simulink model "global_noise"  (R2023a)
settings: Solver=VariableStepAuto  StartTime=0.0  StopTime=10  RelTol=1e-3
values from neighbouring files (symbols this model uses):
  Ad = [0 0 0 0 0 0 ... (first row only)    [Project_globale.m]    (also in Project_locale.m)
  Ai = A0    [Project_globale.m]    (also in Project_locale.m)
  Bi = [ 0 ; -9.9453]    [Project_globale.m]    (also in Project_locale.m)
  c = 10/2*min(real(lambda_g))    [Project_globale.m]    (also in Project_locale.m)
  Ci = [708.27 0]    [Project_globale.m]    (also in Project_locale.m)
  F = P*Ci'*R^-1    [Project_globale.m]
  G = diag([1 0 0 0 0 0])    [Project_globale.m]    (also in Project_locale.m)
  K = R^-1*Bi'*P    [Project_globale.m]    (also in Project_locale.m)
  L0 = place(Ai',Ci',[0 -3])'    [Project_globale.m]
  x0 = [3,1]    [Project_globale.m]    (also in Project_locale.m)
settings Model: Creator=Giulia  LastModifiedBy=Giulia

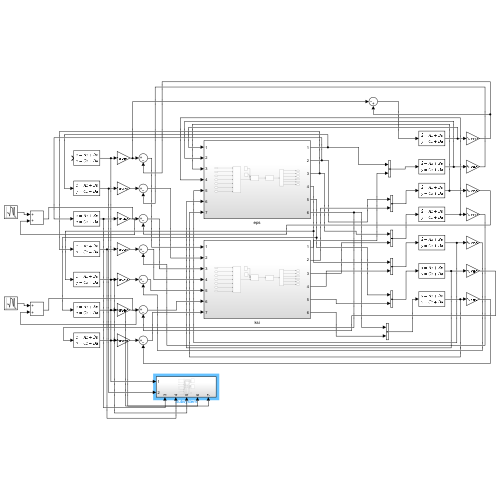
[thumbnail: Simulink's stored preview of the top-level diagram]
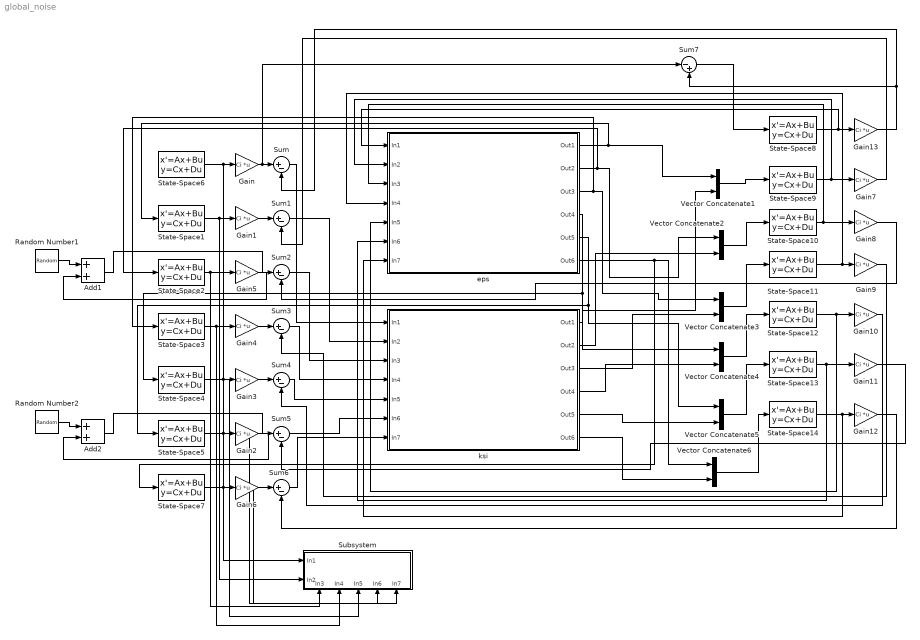
== system global_noise ==
  Add1 : Sum
  Add2 : Sum
  Gain{,1..13} (14 alike) : Gain  Gain=Ci  Multiplication=Matrix(K*u) (u vector)
  Random Number1 : RandomNumber  Variance=10000  SampleTime=0.1
  Random Number2 : RandomNumber  Variance=10000  SampleTime=0.1
  State-Space{1..5,7} (6 alike) : StateSpace  A=Ai  B=c*Bi*K  C=eye(2)  D=zeros(2,2)  InitialCondition=x0  ParameterTunability=Optimized
  State-Space{9..14} (6 alike) : StateSpace  A=Ai  B=[c*Bi*K,-c*F]  C=eye(2)  D=zeros(2,3)  InitialCondition=x0  ParameterTunability=Optimized
  State-Space6 : StateSpace  A=Ai  B=Bi  C=eye(2)  D=zeros(2,1)  InitialCondition=x0  ParameterTunability=Optimized
  State-Space8 : StateSpace  A=Ai  B=-L0  C=eye(2)  D=zeros(2,1)  InitialCondition=x0  ParameterTunability=Optimized
  Subsystem : Subsystem
      settings: PortSchema="{\"entries\":[{\"content\":{\"sides\":[{\"content\":{\"connectorIds\":[\"In1\",\"In2\"]},\"type\":\"ConnectorPlacement.EquallySpacedRectSide\",\"uuid\":\"e5690f60-dfa3-4d24-845c-eb19d446c7ee\"},{\"content\":{\"side\":\"RIGHT\"},\"type\":\"ConnectorPlacement.EquallySpacedRectSide\",\"uuid\":\"a41d9e4a-267d-44ba-a380-b8d8ea4e3cb9\"},{\"content\":{\"side\":\"TOP\"},\"type\":\"ConnectorPlacement.EquallySpacedRectSide\",\"uuid\":\"990e4c72-4654-4e9a-98e4-634db6676fa3\"},{\"content\":{\"connectorIds\":[\"In3\",\"In4\",\"In5\",\"In6\",\"In7\"],\"side\":\"BOTTOM\"},\"type\":\"ConnectorPlacement.EquallySpacedRectSide\",\"uuid\":\"e75a7693-b495-4998-ab10-28f33e3d4652\"}]},\"type\":\"ConnectorPlacement.EquallySpacedConnector\",\"uuid\":\"cc17a25f-dba8-4ee4-98f7-88763bf16359\"}],\"packageUris\":[\"http://schema.mathworks.com/mf0/Connector/R2020b\"],\"version\":\"1.0\"}"
  Sum{,1..6} (7 alike) : Sum  Inputs=|+-
  Sum7 : Sum  Inputs=|-+
  Vector Concatenate{1..6} (6 alike) : Concatenate
  eps : Subsystem
  ksi : Subsystem
  wires:
  ksi/1(Out1) -> Vector Concatenate1/2
  Sum6/1 -> ksi/7(In7)
  Gain/1 -> Sum7/1, Sum/1
  Sum3/1 -> ksi/4(In4)
  Sum2/1 -> ksi/3(In3)
  Sum5/1 -> ksi/6(In6)
  Gain7/1 -> Sum1/2
  Gain9/1 -> Sum3/2
  Sum4/1 -> ksi/5(In5)
  Gain8/1 -> Sum2/2
  Gain13/1 -> Sum7/2, Sum/2
  Gain10/1 -> Sum4/2
  Vector Concatenate6/1 -> State-Space14/1
  Vector Concatenate3/1 -> State-Space11/1
  ksi/2(Out2) -> Vector Concatenate2/2
  ksi/4(Out4) -> Vector Concatenate4/2
  Vector Concatenate2/1 -> State-Space10/1
  ksi/6(Out6) -> Vector Concatenate6/2
  eps/4(Out4) -> State-Space4/1, Vector Concatenate4/1
  eps/5(Out5) -> State-Space5/1, Vector Concatenate5/1
  Gain11/1 -> Sum5/2
  eps/6(Out6) -> State-Space7/1, Vector Concatenate6/1
  State-Space12/1 -> eps/5(In5), Gain10/1
  ksi/3(Out3) -> Vector Concatenate3/2
  eps/2(Out2) -> State-Space2/1, Vector Concatenate2/1
  State-Space8/1 -> eps/1(In1), Gain13/1
  eps/1(Out1) -> State-Space1/1, Vector Concatenate1/1
  State-Space11/1 -> eps/4(In4), Gain9/1
  State-Space13/1 -> eps/6(In6), Gain11/1
  State-Space4/1 -> Subsystem/5(In5), Gain3/1
  Vector Concatenate4/1 -> State-Space12/1
  Gain3/1 -> Sum4/1
  Sum/1 -> ksi/1(In1)
  Sum1/1 -> ksi/2(In2)
  ksi/5(Out5) -> Vector Concatenate5/2
  Vector Concatenate5/1 -> State-Space13/1
  State-Space3/1 -> Subsystem/4(In4), Gain4/1
  Gain1/1 -> Sum1/1
  eps/3(Out3) -> State-Space3/1, Vector Concatenate3/1
  Vector Concatenate1/1 -> State-Space9/1
  State-Space1/1 -> Subsystem/2(In2), Gain1/1
  State-Space6/1 -> Subsystem/1(In1), Gain/1
  State-Space9/1 -> eps/2(In2), Gain7/1
  Gain12/1 -> Sum6/2
  Sum7/1 -> State-Space8/1
  State-Space14/1 -> eps/7(In7), Gain12/1
  State-Space10/1 -> Gain8/1, eps/3(In3)
  State-Space2/1 -> Subsystem/3(In3), Gain5/1
  State-Space5/1 -> Subsystem/6(In6), Gain2/1
  Gain4/1 -> Sum3/1
  State-Space7/1 -> Subsystem/7(In7), Gain6/1
  Random Number1/1 -> Add1/1
  Add1/1 -> Sum2/1
  Gain5/1 -> Add1/2
  Random Number2/1 -> Add2/1
  Gain2/1 -> Add2/2
  Add2/1 -> Sum5/1
  Gain6/1 -> Sum6/1

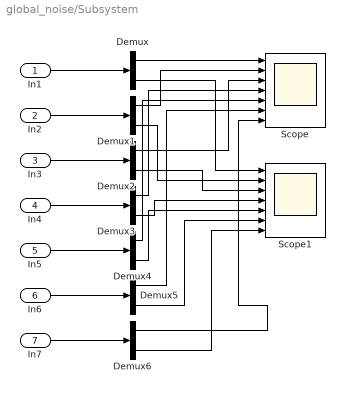
== system global_noise/Subsystem ==
  In1 : Inport
  In2 : Inport  Port=2
  In3 : Inport  Port=3
  In4 : Inport  Port=4
  In5 : Inport  Port=5
  In6 : Inport  Port=6
  In7 : Inport  Port=7
  Demux{,1..6} (7 alike) : Demux  Outputs=2
  Scope : Scope  NumInputPorts=7
  Scope1 : Scope  NumInputPorts=7
  wires:
  In1/1 -> Demux/1
  In2/1 -> Demux1/1
  In3/1 -> Demux2/1
  In4/1 -> Demux3/1
  In5/1 -> Demux4/1
  In6/1 -> Demux5/1
  In7/1 -> Demux6/1
  Demux/1 -> Scope/1
  Demux1/1 -> Scope/2
  Demux2/1 -> Scope/3
  Demux3/1 -> Scope/4
  Demux4/1 -> Scope/5
  Demux5/1 -> Scope/6
  Demux6/1 -> Scope/7
  Demux/2 -> Scope1/1
  Demux1/2 -> Scope1/2
  Demux2/2 -> Scope1/3
  Demux3/2 -> Scope1/4
  Demux4/2 -> Scope1/5
  Demux5/2 -> Scope1/6
  Demux6/2 -> Scope1/7

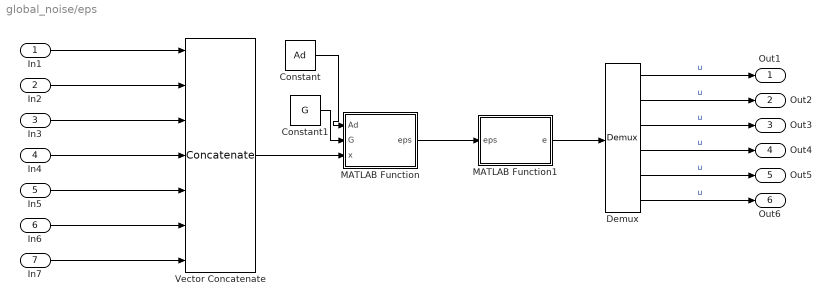
== system global_noise/eps ==
  In1 : Inport
  In2 : Inport  Port=2
  In3 : Inport  Port=3
  In4 : Inport  Port=4
  In5 : Inport  Port=5
  In6 : Inport  Port=6
  In7 : Inport  Port=7
  Constant : Constant  Value=Ad
  Constant1 : Constant  Value=G
  Demux : Demux  Outputs=size(Ad,1)
  MATLAB Function : MATLAB Function  TreatAsAtomicUnit=on
  MATLAB Function1 : MATLAB Function  TreatAsAtomicUnit=on
  Vector Concatenate : Concatenate  NumInputs=7  Mode=Multidimensional array  ConcatenateDimension=2
  Out1 : Outport
  Out2 : Outport  Port=2
  Out3 : Outport  Port=3
  Out4 : Outport  Port=4
  Out5 : Outport  Port=5
  Out6 : Outport  Port=6
  wires:
  MATLAB Function1/1(e) -> Demux/1
  Constant/1 -> MATLAB Function/1(Ad)
  MATLAB Function/1(eps) -> MATLAB Function1/1(eps)
  Constant1/1 -> MATLAB Function/2(G)
  Vector Concatenate/1 -> MATLAB Function/3(x)
  In1/1 -> Vector Concatenate/1
  In2/1 -> Vector Concatenate/2
  In3/1 -> Vector Concatenate/3
  In4/1 -> Vector Concatenate/4
  In5/1 -> Vector Concatenate/5
  In6/1 -> Vector Concatenate/6
  In7/1 -> Vector Concatenate/7
  Demux/1 -> Out1/1  "u"
  Demux/2 -> Out2/1  "u"
  Demux/3 -> Out3/1  "u"
  Demux/4 -> Out4/1  "u"
  Demux/5 -> Out5/1  "u"
  Demux/6 -> Out6/1  "u"

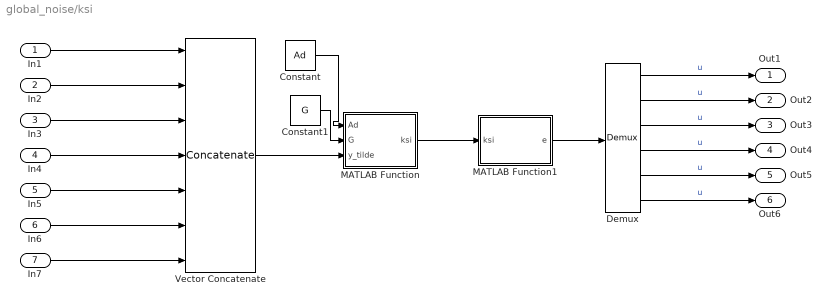
== system global_noise/ksi ==
  In1 : Inport
  In2 : Inport  Port=2
  In3 : Inport  Port=3
  In4 : Inport  Port=4
  In5 : Inport  Port=5
  In6 : Inport  Port=6
  In7 : Inport  Port=7
  Constant : Constant  Value=Ad
  Constant1 : Constant  Value=G
  Demux : Demux  Outputs=size(Ad,1)
  MATLAB Function : MATLAB Function  TreatAsAtomicUnit=on
  MATLAB Function1 : MATLAB Function  TreatAsAtomicUnit=on
  Vector Concatenate : Concatenate  NumInputs=7  Mode=Multidimensional array  ConcatenateDimension=2
  Out1 : Outport
  Out2 : Outport  Port=2
  Out3 : Outport  Port=3
  Out4 : Outport  Port=4
  Out5 : Outport  Port=5
  Out6 : Outport  Port=6
  wires:
  MATLAB Function1/1(e) -> Demux/1
  Constant/1 -> MATLAB Function/1(Ad)
  MATLAB Function/1(ksi) -> MATLAB Function1/1(ksi)
  Constant1/1 -> MATLAB Function/2(G)
  Vector Concatenate/1 -> MATLAB Function/3(y_tilde)
  In1/1 -> Vector Concatenate/1
  In2/1 -> Vector Concatenate/2
  In3/1 -> Vector Concatenate/3
  In4/1 -> Vector Concatenate/4
  In5/1 -> Vector Concatenate/5
  In6/1 -> Vector Concatenate/6
  In7/1 -> Vector Concatenate/7
  Demux/1 -> Out1/1  "u"
  Demux/2 -> Out2/1  "u"
  Demux/3 -> Out3/1  "u"
  Demux/4 -> Out4/1  "u"
  Demux/5 -> Out5/1  "u"
  Demux/6 -> Out6/1  "u"

== matlab function global_noise/eps/MATLAB Function1 ==
  data: eps input; e output
function e = matrix_to_vec(eps)

e=zeros(size(eps,1)*size(eps,2),1);
for i=1:size(eps,2)
    for j=1:size(eps,1)
        e((i-1)*size(eps,1)+j)=eps(j,i);
    end
end

== matlab function global_noise/eps/MATLAB Function ==
  data: Ad input; G input; eps output; x input
function eps = tracking_error(Ad, G, x)

eps=zeros(size(x,1),size(Ad,1));            %2 righe, 6 colonne
for i=1:size(Ad,1)
    sum=zeros(2,1);
    for j=1:size(Ad,1)
        sum=sum+Ad(i,j)*(x(:,1+j)-x(:,1+i));
    end
    sum=sum+G(i,i)*(x(:,1)-x(:,1+i));
    eps(:,i)=sum;
end

== matlab function global_noise/ksi/MATLAB Function ==
  data: Ad input; G input; ksi output; y_tilde input
function ksi = tracking_error(Ad, G, y_tilde)

ksi=zeros(size(y_tilde,1),size(Ad,1));            
for i=1:size(Ad,1)
    sum=0;
    for j=1:size(Ad,1)
        sum=sum+Ad(i,j)*(y_tilde(:,1+j)-y_tilde(:,1+i));
    end
    sum=sum+G(i,i)*(y_tilde(:,1)-y_tilde(:,1+i));
    ksi(:,i)=sum;
end

== matlab function global_noise/ksi/MATLAB Function1 ==
  data: ksi input; e output
function e = matrix_to_vec(ksi)

e=zeros(size(ksi,1)*size(ksi,2),1);
for i=1:size(ksi,2)
    for j=1:size(ksi,1)
        e((i-1)*size(ksi,1)+j)=ksi(j,i);
    end
end
